simulink subsystem "SimscapePlantModels"  (R2023a)
settings: Solver=VariableStepAuto  StartTime=0.0  StopTime=10.0  RelTol=1e-3
undefined symbols (not defined in the file): AxlFL, AxlFR, AxlRL, AxlRR, EM1, EM2, EM3, EM4, PlntDCDCVoltInit, PlntTrnsfrCaseAxlSpdLock, PlntTrnsfrCaseTrqSplitRatio, ThrmBatt, ThrmBatt1, ThrmBatt2, ThrmBatt3, ThrmBatt4, ThrmEM, ThrmEM1, ThrmEM2, ThrmEM3, ThrmEM4, ThrmPwrE
libraries: fl_lib x30, nesl_utility_internal x13, sdl_lib x3, vehdynlibsens x1, nesl_utility x1
(part 2 of 2)

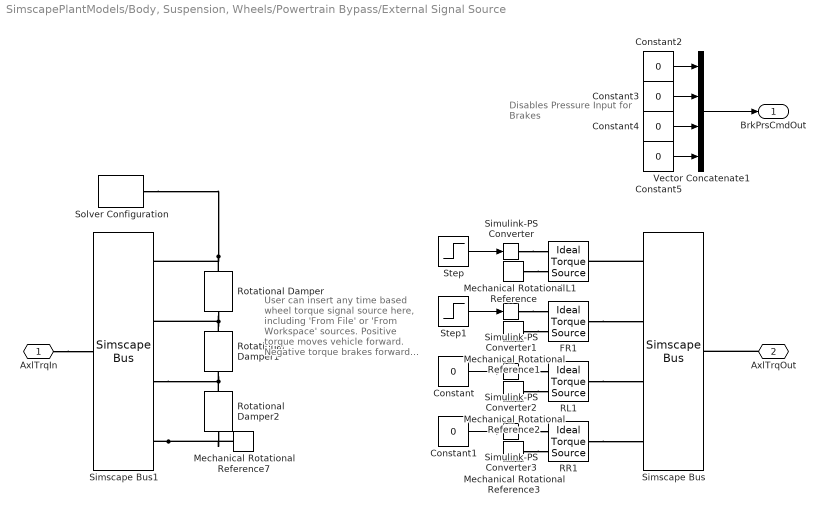
== system SimscapePlantModels/Body, Suspension, Wheels/Powertrain Bypass/External Signal Source ==
  note: User can insert any time based
      | wheel torque signal source here,
      | including 'From File' or 'From
      | Workspace' sources.
      |
      | Positive torque moves vehicle
      | forward.
      | Negative torque brakes forward
      | moving vehicle or moves vehicle
      | in reverse.
  note: Disables Pressure
      | Input for Brakes
  Constant{,1..5} (6 alike) : Constant  Value=0  SampleTime=-1
  FL1 : fl_lib/Mechanical/Mechanical Sources/Ideal Torque Source
  FR1 : fl_lib/Mechanical/Mechanical Sources/Ideal Torque Source
  Mechanical Rotational Reference{,1..3,7} (5 alike) : fl_lib/Mechanical/Rotational Elements/Mechanical Rotational Reference
  RL1 : fl_lib/Mechanical/Mechanical Sources/Ideal Torque Source
  RR1 : fl_lib/Mechanical/Mechanical Sources/Ideal Torque Source
  Rotational Damper : sdl_lib/Couplings & Drives/Springs & Dampers/Rotational Damper  D=1e5 N*m*s/rad  enable_faults=simscape.enum.onoff.off  b_fault=100 N*m*s/rad  temporal_fault=simscape.enum.onoff.off  fault_time=5 s  shock_fault=simscape.enum.onoff.off  acceleration_limit=100 rad/s^2  shock_limit=1  report_fault=simscape.enum.assert.action.none  thermal_port=simscape.enum.thermaleffects.omit  thermal_mass=50 kJ/K  temperature_specify=off  temperature_priority=High  temperature=300 K  temperature_nominal_specify=off  temperature_nominal_unit=K  temperature_nominal_value=1
  Rotational Damper1 : sdl_lib/Couplings & Drives/Springs & Dampers/Rotational Damper  D=1e5 N*m*s/rad  enable_faults=simscape.enum.onoff.off  b_fault=100 N*m*s/rad  temporal_fault=simscape.enum.onoff.off  fault_time=5 s  shock_fault=simscape.enum.onoff.off  acceleration_limit=100 rad/s^2  shock_limit=1  report_fault=simscape.enum.assert.action.none  thermal_port=simscape.enum.thermaleffects.omit  thermal_mass=50 kJ/K  temperature_specify=off  temperature_priority=High  temperature=300 K  temperature_nominal_specify=off  temperature_nominal_unit=K  temperature_nominal_value=1
  Rotational Damper2 : sdl_lib/Couplings & Drives/Springs & Dampers/Rotational Damper  D=1e5 N*m*s/rad  enable_faults=simscape.enum.onoff.off  b_fault=100 N*m*s/rad  temporal_fault=simscape.enum.onoff.off  fault_time=5 s  shock_fault=simscape.enum.onoff.off  acceleration_limit=100 rad/s^2  shock_limit=1  report_fault=simscape.enum.assert.action.none  thermal_port=simscape.enum.thermaleffects.omit  thermal_mass=50 kJ/K  temperature_specify=off  temperature_priority=High  temperature=300 K  temperature_nominal_specify=off  temperature_nominal_unit=K  temperature_nominal_value=1
  Simscape Bus : SimscapeBus  HierarchyStrings=AxlFL;AxlFR;AxlRL;AxlRR
  Simscape Bus1 : SimscapeBus  HierarchyStrings=AxlFL;AxlFR;AxlRL;AxlRR
  Simulink-PS Converter{,1..3} (4 alike) : nesl_utility_internal/Simulink-PS Converter  PhysicalDomain=network_engine_domain  SubClassName=ps_input  LeftPortType=input  RightPortType=output  PseudoPeriodic=off  Frequencies=[]  NoiseDistribution=none  NoiseParameters=[]  Unit=1  AffineConversion=off  FilteringAndDerivatives=provide  SimscapeFilterOrder=1  InputFilterTimeConstant=0.001  UdotUserProvided=0
  Solver Configuration : nesl_utility_internal/Solver Configuration  PhysicalDomain=network_engine_domain  SubClassName=solver  LeftPortType=input  RightPortType=generic  Tones=[]  Harmonics=[]  SimulateNoise=off  Profile=off  UseLocalSampling=off  EnableSwitchedLinearOptims=on  FrequencyDomain=off  UseCCode=off  RelTol=0.001  AbsTol=0.001  MinStep=1e-09  ToWorkspace=off  RevertToSquareIcSolve=off  NumHomotopyIterations=100  PhasorMode=off  PhasorModeNumHarmonics=1  ConsistencySolver=NEWTON_XTOL_AFTER_FTOL  IndexReductionMethod=DerivativeReplacement  DoDC=off  ResidualTolerance=1e-09  ConsistencyTolSource=GLOBAL  ConsistencyAbsTol=0.001  ConsistencyRelTol=0.001  ConsistencyTolFactor=0.001  UseLocalSolver=off  LocalSolverChoice=NE_BACKWARD_EULER_ADVANCER  ResolveIndetEquations=on  FunctionEvalNumThread=1  LocalSolverSampleTime=0.001  DoFixedCost=off  MaxNonlinIter=3  MaxModeIter=2  ComputeImpulses=off  ImpulseIterations=2  LinearAlgebra=auto  LinearAlgebraNumThread=0  EquationFormulation=NE_TIME_EF  DelaysMemoryBudget=1024  AutomaticFiltering=on  FilteringTimeConstant=0.001  PartitionStorageMethod=AS_NEEDED  PartitionMemoryBudget=1024  PartitionMethod=ROBUST
  Step : Step  After=100  SampleTime=0
  Step1 : Step  After=100  SampleTime=0
  Vector Concatenate1 : Concatenate  NumInputs=4
  AxlTrqIn : PMIOPort  Side=Left
  AxlTrqOut : PMIOPort  Port=2  Side=Right
  BrkPrsCmdOut : Outport
  wires:
  Constant2/1 -> Vector Concatenate1/1
  Constant3/1 -> Vector Concatenate1/2
  Constant4/1 -> Vector Concatenate1/3
  Vector Concatenate1/1 -> BrkPrsCmdOut/1
  Constant5/1 -> Vector Concatenate1/4
  Step1/1 -> Simulink-PS Converter1/1
  Step/1 -> Simulink-PS Converter/1
  Constant1/1 -> Simulink-PS Converter3/1
  Constant/1 -> Simulink-PS Converter2/1
  connections:
  Rotational Damper/LConn1 -- Simscape Bus1/LConn1 -- Solver Configuration/RConn1
  Rotational Damper2/LConn1 -- Simscape Bus1/LConn3 -- Rotational Damper1/RConn1
  Simscape Bus1/LConn4 -- Rotational Damper2/RConn1 -- Mechanical Rotational Reference7/LConn1
  Rotational Damper1/LConn1 -- Rotational Damper/RConn1 -- Simscape Bus1/LConn2
  Simulink-PS Converter3/RConn1 -- RR1/RConn1
  AxlTrqOut/RConn1 -- Simscape Bus/RConn1
  RR1/LConn1 -- Simscape Bus/LConn4
  Mechanical Rotational Reference1/LConn1 -- FR1/RConn2
  FR1/LConn1 -- Simscape Bus/LConn2
  AxlTrqIn/RConn1 -- Simscape Bus1/RConn1
  Simulink-PS Converter2/RConn1 -- RL1/RConn1
  RL1/LConn1 -- Simscape Bus/LConn3
  Mechanical Rotational Reference/LConn1 -- FL1/RConn2
  Simulink-PS Converter/RConn1 -- FL1/RConn1
  Mechanical Rotational Reference3/LConn1 -- RR1/RConn2
  Simscape Bus/LConn1 -- FL1/LConn1
  Simulink-PS Converter1/RConn1 -- FR1/RConn1
  Mechanical Rotational Reference2/LConn1 -- RL1/RConn2

== system SimscapePlantModels/Body, Suspension, Wheels/Powertrain Bypass/Pass Through ==
  BrkPrsCmdIn : Inport
  AxlTrqIn : PMIOPort  Side=Left
  AxlTrqOut : PMIOPort  Port=2  Side=Right
  BrkPrsCmdOut : Outport
  wires:
  BrkPrsCmdIn/1 -> BrkPrsCmdOut/1
  connections:
  AxlTrqOut/RConn1 -- AxlTrqIn/RConn1

== system SimscapePlantModels/Drivetrain/Drivetrain Layout/AxlTrqFL ==
  Ideal Torque Sensor : fl_lib/Mechanical/Mechanical Sensors/Ideal Torque Sensor
  PS-Simulink Converter : nesl_utility_internal/PS-Simulink Converter  PhysicalDomain=network_engine_domain  SubClassName=ps_output  LeftPortType=input  RightPortType=output  PseudoPeriodic=off  Frequencies=[]  VectorFormat=inherit  Unit=inherit  AffineConversion=off
  R : PMIOPort  Side=Left
  C : PMIOPort  Port=2  Side=Right
  Trq : Outport
  wires:
  PS-Simulink Converter/1 -> Trq/1
  connections:
  Ideal Torque Sensor/LConn1 -- R/RConn1
  Ideal Torque Sensor/RConn1 -- C/RConn1
  PS-Simulink Converter/LConn1 -- Ideal Torque Sensor/RConn2

== system SimscapePlantModels/Drivetrain/Drivetrain Layout/AxlTrqFR ==
  Ideal Torque Sensor : fl_lib/Mechanical/Mechanical Sensors/Ideal Torque Sensor
  PS-Simulink Converter : nesl_utility_internal/PS-Simulink Converter  PhysicalDomain=network_engine_domain  SubClassName=ps_output  LeftPortType=input  RightPortType=output  PseudoPeriodic=off  Frequencies=[]  VectorFormat=inherit  Unit=inherit  AffineConversion=off
  R : PMIOPort  Side=Left
  C : PMIOPort  Port=2  Side=Right
  Trq : Outport
  wires:
  PS-Simulink Converter/1 -> Trq/1
  connections:
  PS-Simulink Converter/LConn1 -- Ideal Torque Sensor/RConn2
  Ideal Torque Sensor/RConn1 -- C/RConn1
  Ideal Torque Sensor/LConn1 -- R/RConn1

== system SimscapePlantModels/Drivetrain/Drivetrain Layout/AxlTrqR ==
  Ideal Torque Sensor : fl_lib/Mechanical/Mechanical Sensors/Ideal Torque Sensor
  PS-Simulink Converter : nesl_utility_internal/PS-Simulink Converter  PhysicalDomain=network_engine_domain  SubClassName=ps_output  LeftPortType=input  RightPortType=output  PseudoPeriodic=off  Frequencies=[]  VectorFormat=inherit  Unit=inherit  AffineConversion=off
  R : PMIOPort  Side=Left
  C : PMIOPort  Port=2  Side=Right
  Trq : Outport
  wires:
  PS-Simulink Converter/1 -> Trq/1
  connections:
  PS-Simulink Converter/LConn1 -- Ideal Torque Sensor/RConn2
  Ideal Torque Sensor/RConn1 -- C/RConn1
  Ideal Torque Sensor/LConn1 -- R/RConn1

== system SimscapePlantModels/Drivetrain/Drivetrain Layout/AxlTrqRL ==
  Ideal Torque Sensor : fl_lib/Mechanical/Mechanical Sensors/Ideal Torque Sensor
  PS-Simulink Converter : nesl_utility_internal/PS-Simulink Converter  PhysicalDomain=network_engine_domain  SubClassName=ps_output  LeftPortType=input  RightPortType=output  PseudoPeriodic=off  Frequencies=[]  VectorFormat=inherit  Unit=inherit  AffineConversion=off
  R : PMIOPort  Side=Left
  C : PMIOPort  Port=2  Side=Right
  Trq : Outport
  wires:
  PS-Simulink Converter/1 -> Trq/1
  connections:
  Ideal Torque Sensor/LConn1 -- R/RConn1
  Ideal Torque Sensor/RConn1 -- C/RConn1
  PS-Simulink Converter/LConn1 -- Ideal Torque Sensor/RConn2

== system SimscapePlantModels/Drivetrain/Drivetrain Layout/Axle Interconnect ==
  SplitRatio : Inport
  Lockup : Inport  Port=2
  No Interconnect : Subsystem  VariantControl=No Interconnect
  Transfer Case : Subsystem  VariantControl=Transfer Case  ReferencedSubsystem=TransferCaseSSC
  FrntDiffrntlTrq : PMIOPort  Side=Left
  DriveshftTrq : PMIOPort  Port=2  Side=Left
  RearDiffrntlTrq : PMIOPort  Port=3  Side=Left

== system SimscapePlantModels/Drivetrain/Drivetrain Layout/DriveshftTrq Routing ==
  Four Actuator AWD : Subsystem  VariantControl=Four Actuator AWD  ReferencedSubsystem=FourActuatorAWDSSC
  One Actuator AWD : Subsystem  VariantControl=One Actuator AWD  ReferencedSubsystem=OneActuatorAWDSSC
  One Actuator FWD : Subsystem  VariantControl=One Actuator FWD  ReferencedSubsystem=OneActuatorFWDSSC
  One Actuator RWD : Subsystem  VariantControl=One Actuator RWD  ReferencedSubsystem=OneActuatorRWDSSC
  Three Actuator AWD Dual EM Front : Subsystem  VariantControl=Three Actuator AWD Dual EM Front  ReferencedSubsystem=ThreeActuatorAWD2EMFrontSSC
  Three Actuator AWD Dual EM Rear : Subsystem  VariantControl=Three Actuator AWD Dual EM Rear  ReferencedSubsystem=ThreeActuatorAWD2EMRearSSC
  Two Actuator AWD : Subsystem  VariantControl=Two Actuator AWD  ReferencedSubsystem=TwoActuatorAWDSSC
  DriveshftTrq : PMIOPort  Side=Left
  FrntDiffrntlTrq : PMIOPort  Port=2  Side=Right
  TrnsfrCaseFrntTrq : PMIOPort  Port=3  Side=Right
  TrnsfrCaseTrq : PMIOPort  Port=4  Side=Right
  TrnsfrCaseRearTrq : PMIOPort  Port=5  Side=Right
  RearDiffrntlTrq : PMIOPort  Port=6  Side=Right
  DriveshftSpd : Outport  VectorParamsAs1DForOutWhenUnconnected=off

== system SimscapePlantModels/Drivetrain/Drivetrain Layout/Front Axle ==
  Prs1 : Inport
  Prs2 : Inport  Port=2
  Dual EM Drive Front : Subsystem  VariantControl=Dual EM Drive Front  ReferencedSubsystem=DualEMDriveFrontSSC
  Limited Slip Differential : Subsystem  VariantControl=Limited Slip Differential  ReferencedSubsystem=LimitedSlipDifferentialSSC
  No Differential : Subsystem  VariantControl=No Differential  ReferencedSubsystem=NoDifferentialFrontSSC
  Open Differential : Subsystem  VariantControl=Open Differential  ReferencedSubsystem=OpenDifferentialSSC
  DriveshftTrq : PMIOPort  Side=Left
  AxlTrqFL : PMIOPort  Port=2  Side=Right
  AxlTrqFR : PMIOPort  Port=3  Side=Right
  Info : Outport
  DriveshftSpd : Outport  Port=2
  Axl1Spd : Outport  Port=3
  Axl2Spd : Outport  Port=4

== system SimscapePlantModels/Drivetrain/Drivetrain Layout/Rear Axle ==
  Prs1 : Inport
  Prs2 : Inport  Port=2
  Dual EM Rear 3EM : Subsystem  VariantControl=Dual EM Rear 3EM  ReferencedSubsystem=DualEMDriveRear3EMSSC
  Dual EM Rear 4EM : Subsystem  VariantControl=Dual EM Rear 4EM  ReferencedSubsystem=DualEMDriveRear4EMSSC
  Limited Slip Differential : Subsystem  VariantControl=Limited Slip Differential  ReferencedSubsystem=LimitedSlipDifferential2SSC
  No Differential : Subsystem  VariantControl=No Differential  ReferencedSubsystem=NoDifferentialRearSSC
  Open Differential : Subsystem  VariantControl=Open Differential  ReferencedSubsystem=OpenDifferential2SSC
  DriveshftTrq : PMIOPort  Side=Left
  AxlTrqRL : PMIOPort  Port=2  Side=Right
  AxlTrqRR : PMIOPort  Port=3  Side=Right
  Info : Outport
  DriveshftSpd : Outport  Port=2
  Axl1Spd : Outport  Port=3
  Axl2Spd : Outport  Port=4

== system SimscapePlantModels/Drivetrain/Transmission and Actuators/Conventional Vehicle ==
  note: Copyright 2021 The MathWorks, Inc.
  GearCmd : Inport
  Bus Creator : BusCreator  Inputs=3
  Constant : Constant  Value=0  SampleTime=-1
  Inertia1 : fl_lib/Mechanical/Rotational Elements/Inertia  inertia=PlntEngInertia kg*m^2  num_ports=foundation.enum.numPorts2.two  w_specify=off  w_priority=High  w=0 rad/s  w_nominal_specify=off  w_nominal_unit=rad/s  w_nominal_value=1  t_specify=off  t_priority=None  t=0 N*m  t_nominal_specify=off  t_nominal_unit=N*m  t_nominal_value=1
      settings: InternalSimscapePortConfiguration="{\"Bottom\":[],\"Left\":[{\"id\":\"I\",\"label\":\"\",\"type\":\"foundation.mechanical.rotational.rotational\"}],\"Right\":[{\"id\":\"J\",\"label\":\"\",\"type\":\"foundation.mechanical.rotational.rotational\"}],\"Top\":[]}"
  Simscape Bus1 : SimscapeBus  HierarchyStrings=DriveshftTrq1
  Spd Sensor : Subsystem
  Transmission : Subsystem  Variant=on  VariantControlMode=label  VariantControl=1  LabelModeActiveChoice=Ideal Fixed Gear Transmission
  DriveshftTrq : PMIOPort  Side=Right
  EngTrq : PMIOPort  Port=2  Side=Left
  Info : Outport
  EngSpd : Outport  Port=2
  wires:
  Constant/1 -> Bus Creator/1  "Cltch1State"
  Transmission/2(Info) -> Bus Creator/3  "TransInfo"
  Transmission/1(Cltch2State) -> Bus Creator/2  "Cltch2State"
  GearCmd/1 -> Transmission/1(GearCmd)
  Bus Creator/1 -> Info/1
  Spd Sensor/1(w) -> EngSpd/1
  connections:
  DriveshftTrq/RConn1 -- Simscape Bus1/RConn1
  Inertia1/LConn1 -- Transmission/LConn1
  Spd Sensor/LConn1 -- EngTrq/RConn1 -- Inertia1/RConn1
  Simscape Bus1/LConn1 -- Transmission/RConn1

== system SimscapePlantModels/Electrical System/Electrical System/Battery System ==
  P_Acc : Inport
  BMS : Inport  Port=2
  AmbTemp : Inport  Port=3
  Detailed Battery : Subsystem  VariantControl=Detailed Battery  ReferencedSubsystem=DetailedBatteryModel
  Mapped Battery : Subsystem  VariantControl=Mapped Battery  ReferencedSubsystem=BatteryMappedSSC
  + : PMIOPort  Side=Right
  - : PMIOPort  Port=2  Side=Right
  ThrmBatt : PMIOPort  Port=3  Side=Right
  BattSoc : Outport  VectorParamsAs1DForOutWhenUnconnected=off
  BattVolt : Outport  Port=2  VectorParamsAs1DForOutWhenUnconnected=off
  BattCurr : Outport  Port=3  VectorParamsAs1DForOutWhenUnconnected=off
  BMSSensors : Outport  Port=4  VectorParamsAs1DForOutWhenUnconnected=off

== system SimscapePlantModels/Electrical System/Electrical System/DC-DC Converter ==
  DC-DC Converter : Subsystem  VariantControl=DC-DC Converter  ReferencedSubsystem=DCDCConverterSSC
  No DC-DC Converter : Subsystem  VariantControl=No DC-DC Converter  ReferencedSubsystem=NoDCDCConverterSSC
  1+ : PMIOPort  Side=Left
  2+ : PMIOPort  Port=2  Side=Right
  1- : PMIOPort  Port=3  Side=Left
  2- : PMIOPort  Port=4  Side=Right
  H : PMIOPort  Port=5  Side=Right
  Vref : PMIOPort  Port=6  Side=Left

== system SimscapePlantModels/Electrical System/Electrical System/Electric Machines ==
  EMTrqCmd : Inport
  1EM : Subsystem  VariantControl=1EM
  2EM : Subsystem  VariantControl=2EM
  3EM : Subsystem  VariantControl=3EM
  4EM : Subsystem  VariantControl=4EM
  + : PMIOPort  Side=Left
  EM : PMIOPort  Port=2  Side=Right
  - : PMIOPort  Port=3  Side=Left
  ThrmEM : PMIOPort  Port=4  Side=Right
  EMTrq : Outport
  EMPwrElec : Outport  Port=2

== system SimscapePlantModels/Electrical System/Electrical System 1EM/Battery System ==
  note: 1) Add Subsystem or Model blocks as valid variant choices.
      | 2) You cannot connect blocks at this level. At simulation, connectivity is automatically
      | determined, based on the active variant and port name matching.
  P_Acc : Inport
  BMS : Inport  Port=2
  AmbTemp : Inport  Port=3
  Detailed Battery : Subsystem  VariantControl=Detailed Battery  ReferencedSubsystem=DetailedBatteryModel
  Mapped Battery : Subsystem  VariantControl=Mapped Battery  ReferencedSubsystem=BatteryMappedSSC
  + : PMIOPort  Side=Right
  - : PMIOPort  Port=2  Side=Right
  BattSoc : Outport  VectorParamsAs1DForOutWhenUnconnected=off
  BattVolt : Outport  Port=2  VectorParamsAs1DForOutWhenUnconnected=off
  BattCurr : Outport  Port=3  VectorParamsAs1DForOutWhenUnconnected=off
  BMSSensors : Outport  Port=4  VectorParamsAs1DForOutWhenUnconnected=off

== system SimscapePlantModels/Electrical System/Electrical System 1EM/DC-DC Converter ==
  DC-DC Converter : Subsystem  VariantControl=DC-DC Converter  ReferencedSubsystem=DCDCConverterSSC
  No DC-DC Converter : Subsystem  VariantControl=No DC-DC Converter  ReferencedSubsystem=NoDCDCConverterSSC
  1+ : PMIOPort  Side=Left
  2+ : PMIOPort  Port=2  Side=Right
  1- : PMIOPort  Port=3  Side=Left
  2- : PMIOPort  Port=4  Side=Right
  H : PMIOPort  Port=5  Side=Right
  Vref : PMIOPort  Port=6  Side=Left

== system SimscapePlantModels/Electrical System/Electrical System 1EM/Electric Machine 1 ==
  EMTrqCmd : Inport
  Mapped EM : Subsystem  VariantControl=Mapped EM  ReferencedSubsystem=ElectricMachine1SSC
  + : PMIOPort  Side=Left
  - : PMIOPort  Port=2  Side=Left
  R : PMIOPort  Port=3  Side=Right
  H : PMIOPort  Port=4  Side=Right
  EMTrq : Outport  VectorParamsAs1DForOutWhenUnconnected=off
  EMPwrElec : Outport  Port=2  VectorParamsAs1DForOutWhenUnconnected=off

== system SimscapePlantModels/Electrical System/Electrical System 2EM/Battery System ==
  note: 1) Add Subsystem or Model blocks as valid variant choices.
      | 2) You cannot connect blocks at this level. At simulation, connectivity is automatically
      | determined, based on the active variant and port name matching.
  P_Acc : Inport
  BMS : Inport  Port=2
  AmbTemp : Inport  Port=3
  Detailed Battery : Subsystem  VariantControl=Detailed Battery  ReferencedSubsystem=DetailedBatteryModel
  Mapped Battery : Subsystem  VariantControl=Mapped Battery  ReferencedSubsystem=BatteryMappedSSC
  + : PMIOPort  Side=Right
  - : PMIOPort  Port=2  Side=Right
  BattSoc : Outport  VectorParamsAs1DForOutWhenUnconnected=off
  BattVolt : Outport  Port=2  VectorParamsAs1DForOutWhenUnconnected=off
  BattCurr : Outport  Port=3  VectorParamsAs1DForOutWhenUnconnected=off
  BMSSensors : Outport  Port=4  VectorParamsAs1DForOutWhenUnconnected=off

== system SimscapePlantModels/Electrical System/Electrical System 2EM/DC-DC Converter ==
  DC-DC Converter : Subsystem  VariantControl=DC-DC Converter  ReferencedSubsystem=DCDCConverterSSC
  No DC-DC Converter : Subsystem  VariantControl=No DC-DC Converter  ReferencedSubsystem=NoDCDCConverterSSC
  1+ : PMIOPort  Side=Left
  2+ : PMIOPort  Port=2  Side=Right
  1- : PMIOPort  Port=3  Side=Left
  2- : PMIOPort  Port=4  Side=Right
  H : PMIOPort  Port=5  Side=Right
  Vref : PMIOPort  Port=6  Side=Left

== system SimscapePlantModels/Electrical System/Electrical System 2EM/Electric Machine 1 ==
  EMTrqCmd : Inport
  Mapped EM : Subsystem  VariantControl=Mapped EM  ReferencedSubsystem=ElectricMachine1SSC
  + : PMIOPort  Side=Left
  - : PMIOPort  Port=2  Side=Left
  R : PMIOPort  Port=3  Side=Right
  H : PMIOPort  Port=4  Side=Right
  EMTrq : Outport  VectorParamsAs1DForOutWhenUnconnected=off
  EMPwrElec : Outport  Port=2  VectorParamsAs1DForOutWhenUnconnected=off

== system SimscapePlantModels/Electrical System/Electrical System 2EM/Electric Machine 2 ==
  EMTrqCmd : Inport
  Mapped EM : Subsystem  VariantControl=Mapped EM  ReferencedSubsystem=ElectricMachine2SSC
  + : PMIOPort  Side=Left
  - : PMIOPort  Port=2  Side=Left
  R : PMIOPort  Port=3  Side=Right
  H : PMIOPort  Port=4  Side=Right
  EMTrq : Outport  VectorParamsAs1DForOutWhenUnconnected=off
  EMPwrElec : Outport  Port=2  VectorParamsAs1DForOutWhenUnconnected=off

== system SimscapePlantModels/Sensors/Sensors/IMU Sensor ==
  VehFdbk : Inport
  Bus Creator1 : BusCreator  Inputs=2
  Bus Selector : BusSelector  OutputSignals=BdyFrm.Cg.Acc.ax,BdyFrm.Cg.Acc.ay,BdyFrm.Cg.Acc.az  OutputAsBus=on
  Bus Selector1 : BusSelector  OutputSignals=BdyFrm.Cg.AngVel.p,BdyFrm.Cg.AngVel.q,BdyFrm.Cg.AngVel.r  OutputAsBus=on
  Bus Selector2 : BusSelector  OutputSignals=BdyFrm.Cg.AngAcc.pdot,BdyFrm.Cg.AngAcc.qdot,BdyFrm.Cg.AngAcc.rdot  OutputAsBus=on
  Bus to Vector : BusToVector
  Bus to Vector1 : BusToVector
  Bus to Vector2 : BusToVector
  Constant : Constant  Value=[0,0,0]
  Constant1 : Constant  Value=[0,0,9.81]
  Three-axis Inertial Measurement Unit : vehdynlibsens/Three-axis Inertial Measurement Unit  units=Metric (MKS)  imu=[0 0 0]  i_Ts=0  dtype_a=off  w_a=190  z_a=0.707  a_sf_cc=[1 0 0; 0 1 0; 0 0 1]  a_bias=[0 0 0]  a_sat="[-inf  -inf  -inf  inf inf inf]"  dtype_g=off  w_g=190  z_g=0.707  g_sf_cc=[1 0 0; 0 1 0; 0 0 1]  g_bias=[0 0 0]  g_sens=[0 0 0]  g_sat="[-inf  -inf  -inf  inf inf inf]"  i_rand=on  i_seeds=[23093 23094 23095 23096 23097 23098]  i_pow=[0.001 0.001 0.001 0.0001 0.0001 0.0001]  aMode=2
  Unit Conversion : UnitConversion
  IMU : Outport
  wires:
  VehFdbk/1 -> Bus Selector/1, Bus Selector1/1, Bus Selector2/1
  Constant1/1 -> Three-axis Inertial Measurement Unit/5
  Bus to Vector/1 -> Unit Conversion/1
  Bus Selector1/1 -> Bus to Vector1/1
  Bus to Vector1/1 -> Three-axis Inertial Measurement Unit/2
  Bus Selector/1 -> Bus to Vector/1
  Bus to Vector2/1 -> Three-axis Inertial Measurement Unit/3
  Three-axis Inertial Measurement Unit/1 -> Bus Creator1/1  "Acc"
  Bus Creator1/1 -> IMU/1  "IMU"
  Bus Selector2/1 -> Bus to Vector2/1
  Constant/1 -> Three-axis Inertial Measurement Unit/4
  Three-axis Inertial Measurement Unit/2 -> Bus Creator1/2  "pqr"
  Unit Conversion/1 -> Three-axis Inertial Measurement Unit/1

== system SimscapePlantModels/Sensors/Sensors/No IMU Sensor ==
  VehFdbk : Inport
  Bus Creator1 : BusCreator  Inputs=2
  Constant : Constant  Value=zeros(3,1)
  Constant1 : Constant  Value=zeros(3,1)
  Terminator : Terminator
  IMU : Outport
  wires:
  VehFdbk/1 -> Terminator/1
  Constant1/1 -> Bus Creator1/2  "pqr"
  Bus Creator1/1 -> IMU/1  "IMU"
  Constant/1 -> Bus Creator1/1  "Acc"

== system SimscapePlantModels/Thermal/Electrical Cooling/No Thermal Effect ==
  BMSSensors : Inport
  VehBody : Inport  Port=2
  Constant : Constant  Value=0  SampleTime=-1
  Constant1 : Constant  Value=0  SampleTime=-1
  Simscape Bus : SimscapeBus  HierarchyStrings=ThrmEM;ThrmBatt;ThrmPwrE
  Simscape Bus1 : SimscapeBus  HierarchyStrings=ThrmEM4;ThrmEM3;ThrmEM2;ThrmEM1
  Simscape Bus2 : SimscapeBus  HierarchyStrings=ThrmBatt4;ThrmBatt3;ThrmBatt2;ThrmBatt1
  Simscape Bus3 : SimscapeBus  HierarchyStrings=ThrmPwrE1
  Temperature Source{,1..8} (9 alike) : fl_lib/Thermal/Thermal Sources/Temperature Source  temperature=EnvAirTemp K
  Terminator : Terminator
  Terminator1 : Terminator
  ThrmElec : PMIOPort  Side=Left
  Out Bus Element : Outport  PortName=Thermal  Element=EPumpPwr
  Out Bus Element1 : Outport  PortName=Thermal  Element=CoolTemp
  wires:
  VehBody/1 -> Terminator1/1
  BMSSensors/1 -> Terminator/1
  Constant/1 -> Out Bus Element/1
  Constant1/1 -> Out Bus Element1/1
  connections:
  Temperature Source3/LConn1 -- Simscape Bus1/LConn4
  Simscape Bus/LConn2 -- Simscape Bus2/RConn1
  Simscape Bus1/RConn1 -- Simscape Bus/LConn1
  ThrmElec/RConn1 -- Simscape Bus/RConn1
  Temperature Source7/LConn1 -- Simscape Bus2/LConn4
  Temperature Source6/LConn1 -- Simscape Bus2/LConn3
  Temperature Source4/LConn1 -- Simscape Bus2/LConn1
  Temperature Source5/LConn1 -- Simscape Bus2/LConn2
  Temperature Source2/LConn1 -- Simscape Bus1/LConn3
  Temperature Source1/LConn1 -- Simscape Bus1/LConn2
  Temperature Source/LConn1 -- Simscape Bus1/LConn1
  Temperature Source8/LConn1 -- Simscape Bus3/LConn1
  Simscape Bus/LConn3 -- Simscape Bus3/RConn1

== system SimscapePlantModels/Drivetrain/Drivetrain Layout/Axle Interconnect/No Interconnect ==

== system SimscapePlantModels/Drivetrain/Transmission and Actuators/Conventional Vehicle/Spd Sensor ==
  Ideal Rotational Motion Sensor : fl_lib/Mechanical/Mechanical Sensors/Ideal Rotational Motion Sensor  reference=foundation.enum.MeasurementReference.difference  acceleration_port=false  velocity_port=true  position_port=true  wrap_angle=simscape.enum.onoff.off  offset=0 rad
  Mechanical Rotational Reference : fl_lib/Mechanical/Rotational Elements/Mechanical Rotational Reference
  PS-Simulink Converter : nesl_utility_internal/PS-Simulink Converter  PhysicalDomain=network_engine_domain  SubClassName=ps_output  LeftPortType=input  RightPortType=output  PseudoPeriodic=off  Frequencies=[]  VectorFormat=inherit  Unit=inherit  AffineConversion=off
  R : PMIOPort  Side=Left
  w : Outport
  wires:
  PS-Simulink Converter/1 -> w/1
  connections:
  PS-Simulink Converter/LConn1 -- Ideal Rotational Motion Sensor/RConn2
  Ideal Rotational Motion Sensor/LConn1 -- R/RConn1
  Ideal Rotational Motion Sensor/RConn1 -- Mechanical Rotational Reference/LConn1

== system SimscapePlantModels/Drivetrain/Transmission and Actuators/Conventional Vehicle/Transmission ==
  GearCmd : Inport
  Automatic Transmission With Torque Converter : Subsystem  VariantControl=Automatic Transmission With Torque Converter  ReferencedSubsystem=AutomaticTransmissionWithTorqueConverterSSC
  Ideal Fixed Gear Transmission : Subsystem  VariantControl=Ideal Fixed Gear Transmission  ReferencedSubsystem=IdealFixedGearTransmissionSSC
  EngTrq : PMIOPort  Side=Left
  DriveshftTrq : PMIOPort  Port=2  Side=Right
  Cltch2State : Outport
  Info : Outport  Port=2

== system SimscapePlantModels/Electrical System/Electrical System/Electric Machines/1EM ==
  EMTrqCmd : Inport
  Electric Machine 1 : Subsystem  Variant=on  VariantControlMode=label  LabelModeActiveChoice=Mapped EM
  Simscape Bus : SimscapeBus  HierarchyStrings=EM1
  Simscape Bus1 : SimscapeBus  HierarchyStrings=ThrmEM1
  + : PMIOPort  Side=Left
  EM : PMIOPort  Port=2  Side=Right
  - : PMIOPort  Port=3  Side=Left
  ThrmEM : PMIOPort  Port=4  Side=Right
  EMTrq : Outport
  EMPwrElec : Outport  Port=2
  wires:
  EMTrqCmd/1 -> Electric Machine 1/1(EMTrqCmd)
  Electric Machine 1/2(EMPwrElec) -> EMPwrElec/1  "EMPwrElec"
  Electric Machine 1/1(EMTrq) -> EMTrq/1  "EMTrq"
  connections:
  Simscape Bus/RConn1 -- EM/RConn1
  -/RConn1 -- Electric Machine 1/LConn2
  +/RConn1 -- Electric Machine 1/LConn1
  Electric Machine 1/RConn1 -- Simscape Bus/LConn1
  ThrmEM/RConn1 -- Simscape Bus1/RConn1
  Simscape Bus1/LConn1 -- Electric Machine 1/RConn2

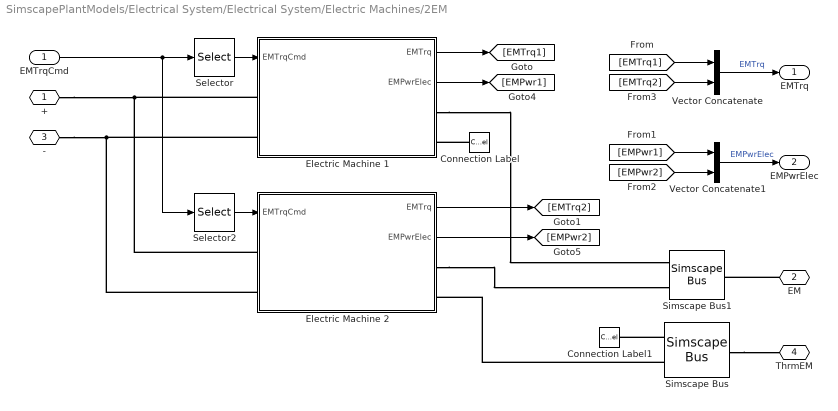
== system SimscapePlantModels/Electrical System/Electrical System/Electric Machines/2EM ==
  EMTrqCmd : Inport
  Connection Label : ConnectionLabel  Label=H1
  Connection Label1 : ConnectionLabel  Label=H1
  Electric Machine 1 : Subsystem  Variant=on  VariantControlMode=label  LabelModeActiveChoice=Mapped EM
  Electric Machine 2 : Subsystem  Variant=on  VariantControlMode=label  LabelModeActiveChoice=Mapped EM
  Selector : Selector  InputPortWidth=2  IndexOptions=Index vector (dialog)  Indices=[1]  OutputSizes=1
  Selector2 : Selector  InputPortWidth=2  IndexOptions=Index vector (dialog)  Indices=[2]  OutputSizes=1
  Simscape Bus : SimscapeBus  HierarchyStrings=ThrmEM1;ThrmEM2
  Simscape Bus1 : SimscapeBus  HierarchyStrings=EM1;EM2
  Vector Concatenate : Concatenate
  Vector Concatenate1 : Concatenate
  + : PMIOPort  Side=Left
  EM : PMIOPort  Port=2  Side=Right
  - : PMIOPort  Port=3  Side=Left
  ThrmEM : PMIOPort  Port=4  Side=Right
  EMTrq : Outport
  EMPwrElec : Outport  Port=2
  wires:
  [EMPwr2] -> Vector Concatenate1/2
  Electric Machine 2/2(EMPwrElec) -> [EMPwr2]
  [EMPwr1] -> Vector Concatenate1/1
  Electric Machine 1/2(EMPwrElec) -> [EMPwr1]
  Electric Machine 2/1(EMTrq) -> [EMTrq2]
  [EMTrq2] -> Vector Concatenate/2
  [EMTrq1] -> Vector Concatenate/1
  Electric Machine 1/1(EMTrq) -> [EMTrq1]
  Selector2/1 -> Electric Machine 2/1(EMTrqCmd)
  Vector Concatenate1/1 -> EMPwrElec/1  "EMPwrElec"
  Vector Concatenate/1 -> EMTrq/1  "EMTrq"
  Selector/1 -> Electric Machine 1/1(EMTrqCmd)
  EMTrqCmd/1 -> Selector/1, Selector2/1
  connections:
  EM/RConn1 -- Simscape Bus1/RConn1
  Electric Machine 2/RConn1 -- Simscape Bus1/LConn2
  Electric Machine 1/RConn1 -- Simscape Bus1/LConn1
  Electric Machine 2/LConn1 -- Electric Machine 1/LConn1 -- +/RConn1
  Electric Machine 2/LConn2 -- Electric Machine 1/LConn2 -- -/RConn1
  Simscape Bus/RConn1 -- ThrmEM/RConn1
  Connection Label/LConn1 -- Electric Machine 1/RConn2
  Simscape Bus/LConn1 -- Connection Label1/LConn1
  Simscape Bus/LConn2 -- Electric Machine 2/RConn2

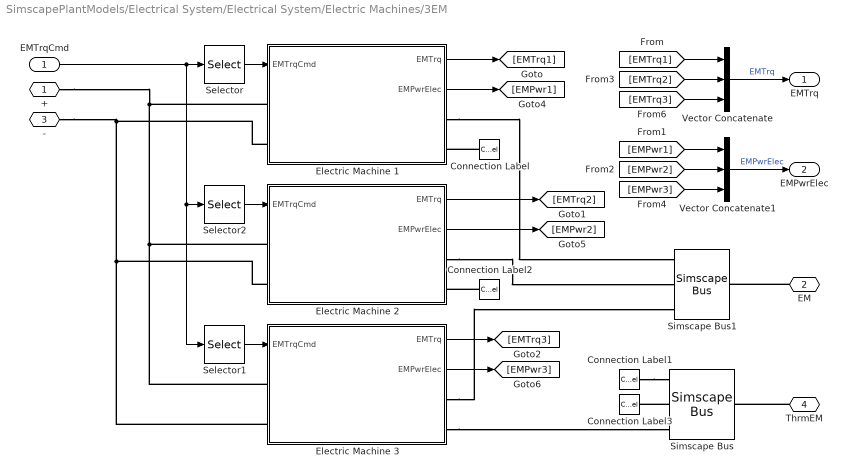
== system SimscapePlantModels/Electrical System/Electrical System/Electric Machines/3EM ==
  EMTrqCmd : Inport
  Connection Label : ConnectionLabel  Label=H1
  Connection Label1 : ConnectionLabel  Label=H1
  Connection Label2 : ConnectionLabel  Label=H2
  Connection Label3 : ConnectionLabel  Label=H2
  Electric Machine 1 : Subsystem  Variant=on  VariantControlMode=label  LabelModeActiveChoice=Mapped EM
  Electric Machine 2 : Subsystem  Variant=on  VariantControlMode=label  LabelModeActiveChoice=Mapped EM
  Electric Machine 3 : Subsystem  Variant=on  VariantControlMode=label  LabelModeActiveChoice=Mapped EM
  Selector : Selector  InputPortWidth=3  IndexOptions=Index vector (dialog)  Indices=[1]  OutputSizes=1
  Selector1 : Selector  InputPortWidth=3  IndexOptions=Index vector (dialog)  Indices=[3]  OutputSizes=1
  Selector2 : Selector  InputPortWidth=3  IndexOptions=Index vector (dialog)  Indices=[2]  OutputSizes=1
  Simscape Bus : SimscapeBus  HierarchyStrings=ThrmEM1;ThrmEM2;ThrmEM3
  Simscape Bus1 : SimscapeBus  HierarchyStrings=EM1;EM2;EM3
  Vector Concatenate : Concatenate  NumInputs=3
  Vector Concatenate1 : Concatenate  NumInputs=3
  + : PMIOPort  Side=Left
  EM : PMIOPort  Port=2  Side=Right
  - : PMIOPort  Port=3  Side=Left
  ThrmEM : PMIOPort  Port=4  Side=Right
  EMTrq : Outport
  EMPwrElec : Outport  Port=2
  wires:
  [EMPwr3] -> Vector Concatenate1/3
  Electric Machine 3/2(EMPwrElec) -> [EMPwr3]
  [EMPwr2] -> Vector Concatenate1/2
  Electric Machine 2/2(EMPwrElec) -> [EMPwr2]
  [EMPwr1] -> Vector Concatenate1/1
  Electric Machine 1/2(EMPwrElec) -> [EMPwr1]
  Electric Machine 3/1(EMTrq) -> [EMTrq3]
  Electric Machine 2/1(EMTrq) -> [EMTrq2]
  [EMTrq3] -> Vector Concatenate/3
  [EMTrq2] -> Vector Concatenate/2
  [EMTrq1] -> Vector Concatenate/1
  Electric Machine 1/1(EMTrq) -> [EMTrq1]
  Selector1/1 -> Electric Machine 3/1(EMTrqCmd)
  Selector2/1 -> Electric Machine 2/1(EMTrqCmd)
  Vector Concatenate1/1 -> EMPwrElec/1  "EMPwrElec"
  Vector Concatenate/1 -> EMTrq/1  "EMTrq"
  EMTrqCmd/1 -> Selector1/1, Selector2/1, Selector/1
  Selector/1 -> Electric Machine 1/1(EMTrqCmd)
  connections:
  Electric Machine 3/RConn1 -- Simscape Bus1/LConn3
  EM/RConn1 -- Simscape Bus1/RConn1
  Electric Machine 2/RConn1 -- Simscape Bus1/LConn2
  Electric Machine 1/RConn1 -- Simscape Bus1/LConn1
  Electric Machine 3/LConn1 -- +/RConn1 -- Electric Machine 1/LConn1 -- Electric Machine 2/LConn1
  Electric Machine 3/LConn2 -- -/RConn1 -- Electric Machine 1/LConn2 -- Electric Machine 2/LConn2
  Connection Label1/LConn1 -- Simscape Bus/LConn1
  Simscape Bus/LConn2 -- Connection Label3/LConn1
  ThrmEM/RConn1 -- Simscape Bus/RConn1
  Connection Label/LConn1 -- Electric Machine 1/RConn2
  Connection Label2/LConn1 -- Electric Machine 2/RConn2
  Electric Machine 3/RConn2 -- Simscape Bus/LConn3

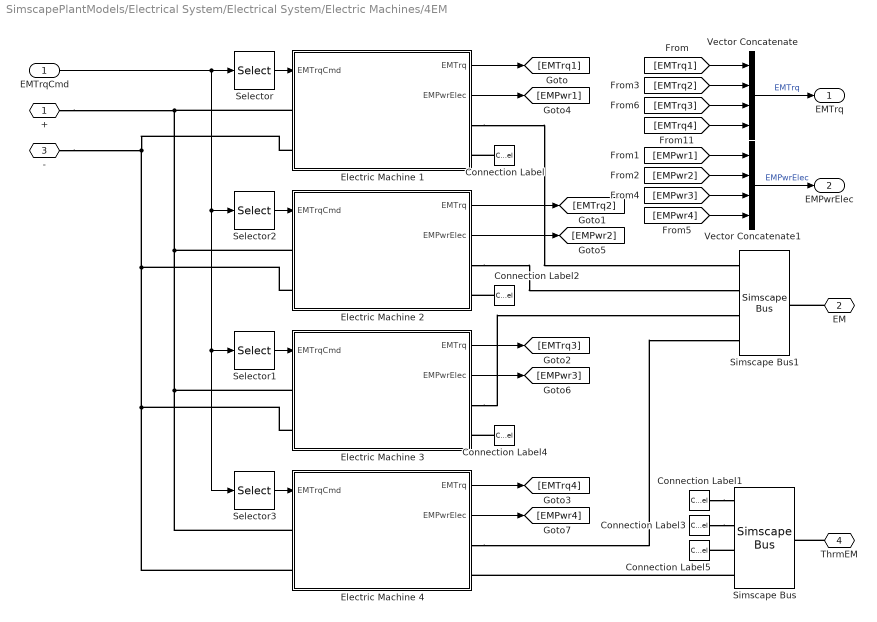
== system SimscapePlantModels/Electrical System/Electrical System/Electric Machines/4EM ==
  EMTrqCmd : Inport
  Connection Label : ConnectionLabel  Label=H1
  Connection Label1 : ConnectionLabel  Label=H1
  Connection Label2 : ConnectionLabel  Label=H2
  Connection Label3 : ConnectionLabel  Label=H2
  Connection Label4 : ConnectionLabel  Label=H3
  Connection Label5 : ConnectionLabel  Label=H3
  Electric Machine 1 : Subsystem  Variant=on  VariantControlMode=label  LabelModeActiveChoice=Mapped EM
  Electric Machine 2 : Subsystem  Variant=on  VariantControlMode=label  LabelModeActiveChoice=Mapped EM
  Electric Machine 3 : Subsystem  Variant=on  VariantControlMode=label  LabelModeActiveChoice=Mapped EM
  Electric Machine 4 : Subsystem  Variant=on  VariantControlMode=label  LabelModeActiveChoice=Mapped EM
  Selector : Selector  InputPortWidth=4  IndexOptions=Index vector (dialog)  Indices=[1]  OutputSizes=1
  Selector1 : Selector  InputPortWidth=4  IndexOptions=Index vector (dialog)  Indices=[3]  OutputSizes=1
  Selector2 : Selector  InputPortWidth=4  IndexOptions=Index vector (dialog)  Indices=[2]  OutputSizes=1
  Selector3 : Selector  InputPortWidth=4  IndexOptions=Index vector (dialog)  Indices=[4]  OutputSizes=1
  Simscape Bus : SimscapeBus  HierarchyStrings=ThrmEM1;ThrmEM2;ThrmEM3;ThrmEM4
  Simscape Bus1 : SimscapeBus  HierarchyStrings=EM1;EM2;EM3;EM4
  Vector Concatenate : Concatenate  NumInputs=4
  Vector Concatenate1 : Concatenate  NumInputs=4
  + : PMIOPort  Side=Left
  EM : PMIOPort  Port=2  Side=Right
  - : PMIOPort  Port=3  Side=Left
  ThrmEM : PMIOPort  Port=4  Side=Right
  EMTrq : Outport
  EMPwrElec : Outport  Port=2
  wires:
  [EMPwr4] -> Vector Concatenate1/4
  Electric Machine 4/2(EMPwrElec) -> [EMPwr4]
  [EMPwr3] -> Vector Concatenate1/3
  Electric Machine 3/2(EMPwrElec) -> [EMPwr3]
  [EMPwr2] -> Vector Concatenate1/2
  Electric Machine 2/2(EMPwrElec) -> [EMPwr2]
  [EMPwr1] -> Vector Concatenate1/1
  Electric Machine 1/2(EMPwrElec) -> [EMPwr1]
  Electric Machine 4/1(EMTrq) -> [EMTrq4]
  Electric Machine 3/1(EMTrq) -> [EMTrq3]
  Electric Machine 2/1(EMTrq) -> [EMTrq2]
  [EMTrq4] -> Vector Concatenate/4
  [EMTrq3] -> Vector Concatenate/3
  [EMTrq2] -> Vector Concatenate/2
  [EMTrq1] -> Vector Concatenate/1
  Electric Machine 1/1(EMTrq) -> [EMTrq1]
  Selector3/1 -> Electric Machine 4/1(EMTrqCmd)
  Selector1/1 -> Electric Machine 3/1(EMTrqCmd)
  Selector2/1 -> Electric Machine 2/1(EMTrqCmd)
  Vector Concatenate1/1 -> EMPwrElec/1  "EMPwrElec"
  Vector Concatenate/1 -> EMTrq/1  "EMTrq"
  Selector/1 -> Electric Machine 1/1(EMTrqCmd)
  EMTrqCmd/1 -> Selector/1, Selector3/1, Selector1/1, Selector2/1
  connections:
  Electric Machine 4/RConn1 -- Simscape Bus1/LConn4
  Electric Machine 3/RConn1 -- Simscape Bus1/LConn3
  EM/RConn1 -- Simscape Bus1/RConn1
  Electric Machine 2/RConn1 -- Simscape Bus1/LConn2
  Electric Machine 1/RConn1 -- Simscape Bus1/LConn1
  Electric Machine 3/LConn1 -- Electric Machine 1/LConn1 -- +/RConn1 -- Electric Machine 2/LConn1 -- Electric Machine 4/LConn1
  Electric Machine 3/LConn2 -- Electric Machine 1/LConn2 -- -/RConn1 -- Electric Machine 2/LConn2 -- Electric Machine 4/LConn2
  Connection Label1/LConn1 -- Simscape Bus/LConn1
  Connection Label3/LConn1 -- Simscape Bus/LConn2
  Simscape Bus/LConn3 -- Connection Label5/LConn1
  Connection Label/LConn1 -- Electric Machine 1/RConn2
  Connection Label2/LConn1 -- Electric Machine 2/RConn2
  ThrmEM/RConn1 -- Simscape Bus/RConn1
  Connection Label4/LConn1 -- Electric Machine 3/RConn2
  Simscape Bus/LConn4 -- Electric Machine 4/RConn2

== system SimscapePlantModels/Electrical System/Electrical System/Electric Machines/1EM/Electric Machine 1 ==
  EMTrqCmd : Inport
  Mapped EM : Subsystem  VariantControl=Mapped EM  ReferencedSubsystem=ElectricMachine1SSC
  + : PMIOPort  Side=Left
  - : PMIOPort  Port=2  Side=Left
  R : PMIOPort  Port=3  Side=Right
  H : PMIOPort  Port=4  Side=Right
  EMTrq : Outport  VectorParamsAs1DForOutWhenUnconnected=off
  EMPwrElec : Outport  Port=2  VectorParamsAs1DForOutWhenUnconnected=off

== system SimscapePlantModels/Electrical System/Electrical System/Electric Machines/2EM/Electric Machine 1 ==
  EMTrqCmd : Inport
  Mapped EM : Subsystem  VariantControl=Mapped EM  ReferencedSubsystem=ElectricMachine1SSC
  + : PMIOPort  Side=Left
  - : PMIOPort  Port=2  Side=Left
  R : PMIOPort  Port=3  Side=Right
  H : PMIOPort  Port=4  Side=Right
  EMTrq : Outport  VectorParamsAs1DForOutWhenUnconnected=off
  EMPwrElec : Outport  Port=2  VectorParamsAs1DForOutWhenUnconnected=off

== system SimscapePlantModels/Electrical System/Electrical System/Electric Machines/2EM/Electric Machine 2 ==
  EMTrqCmd : Inport
  Mapped EM : Subsystem  VariantControl=Mapped EM  ReferencedSubsystem=ElectricMachine2SSC
  + : PMIOPort  Side=Left
  - : PMIOPort  Port=2  Side=Left
  R : PMIOPort  Port=3  Side=Right
  H : PMIOPort  Port=4  Side=Right
  EMTrq : Outport  VectorParamsAs1DForOutWhenUnconnected=off
  EMPwrElec : Outport  Port=2  VectorParamsAs1DForOutWhenUnconnected=off

== system SimscapePlantModels/Electrical System/Electrical System/Electric Machines/3EM/Electric Machine 1 ==
  EMTrqCmd : Inport
  Mapped EM : Subsystem  VariantControl=Mapped EM  ReferencedSubsystem=ElectricMachine1SSC
  + : PMIOPort  Side=Left
  - : PMIOPort  Port=2  Side=Left
  R : PMIOPort  Port=3  Side=Right
  H : PMIOPort  Port=4  Side=Right
  EMTrq : Outport  VectorParamsAs1DForOutWhenUnconnected=off
  EMPwrElec : Outport  Port=2  VectorParamsAs1DForOutWhenUnconnected=off

== system SimscapePlantModels/Electrical System/Electrical System/Electric Machines/3EM/Electric Machine 2 ==
  EMTrqCmd : Inport
  Mapped EM : Subsystem  VariantControl=Mapped EM  ReferencedSubsystem=ElectricMachine2SSC
  + : PMIOPort  Side=Left
  - : PMIOPort  Port=2  Side=Left
  R : PMIOPort  Port=3  Side=Right
  H : PMIOPort  Port=4  Side=Right
  EMTrq : Outport  VectorParamsAs1DForOutWhenUnconnected=off
  EMPwrElec : Outport  Port=2  VectorParamsAs1DForOutWhenUnconnected=off

== system SimscapePlantModels/Electrical System/Electrical System/Electric Machines/3EM/Electric Machine 3 ==
  EMTrqCmd : Inport
  Mapped EM : Subsystem  VariantControl=Mapped EM  ReferencedSubsystem=ElectricMachine3SSC
  + : PMIOPort  Side=Left
  - : PMIOPort  Port=2  Side=Left
  R : PMIOPort  Port=3  Side=Right
  H : PMIOPort  Port=4  Side=Right
  EMTrq : Outport  VectorParamsAs1DForOutWhenUnconnected=off
  EMPwrElec : Outport  Port=2  VectorParamsAs1DForOutWhenUnconnected=off

== system SimscapePlantModels/Electrical System/Electrical System/Electric Machines/4EM/Electric Machine 1 ==
  EMTrqCmd : Inport
  Mapped EM : Subsystem  VariantControl=Mapped EM  ReferencedSubsystem=ElectricMachine1SSC
  + : PMIOPort  Side=Left
  - : PMIOPort  Port=2  Side=Left
  R : PMIOPort  Port=3  Side=Right
  H : PMIOPort  Port=4  Side=Right
  EMTrq : Outport  VectorParamsAs1DForOutWhenUnconnected=off
  EMPwrElec : Outport  Port=2  VectorParamsAs1DForOutWhenUnconnected=off

== system SimscapePlantModels/Electrical System/Electrical System/Electric Machines/4EM/Electric Machine 2 ==
  EMTrqCmd : Inport
  Mapped EM : Subsystem  VariantControl=Mapped EM  ReferencedSubsystem=ElectricMachine2SSC
  + : PMIOPort  Side=Left
  - : PMIOPort  Port=2  Side=Left
  R : PMIOPort  Port=3  Side=Right
  H : PMIOPort  Port=4  Side=Right
  EMTrq : Outport  VectorParamsAs1DForOutWhenUnconnected=off
  EMPwrElec : Outport  Port=2  VectorParamsAs1DForOutWhenUnconnected=off

== system SimscapePlantModels/Electrical System/Electrical System/Electric Machines/4EM/Electric Machine 3 ==
  EMTrqCmd : Inport
  Mapped EM : Subsystem  VariantControl=Mapped EM  ReferencedSubsystem=ElectricMachine3SSC
  + : PMIOPort  Side=Left
  - : PMIOPort  Port=2  Side=Left
  R : PMIOPort  Port=3  Side=Right
  H : PMIOPort  Port=4  Side=Right
  EMTrq : Outport  VectorParamsAs1DForOutWhenUnconnected=off
  EMPwrElec : Outport  Port=2  VectorParamsAs1DForOutWhenUnconnected=off

== system SimscapePlantModels/Electrical System/Electrical System/Electric Machines/4EM/Electric Machine 4 ==
  EMTrqCmd : Inport
  Mapped EM : Subsystem  VariantControl=Mapped EM  ReferencedSubsystem=ElectricMachine4SSC
  + : PMIOPort  Side=Left
  - : PMIOPort  Port=2  Side=Left
  R : PMIOPort  Port=3  Side=Right
  H : PMIOPort  Port=4  Side=Right
  EMTrq : Outport  VectorParamsAs1DForOutWhenUnconnected=off
  EMPwrElec : Outport  Port=2  VectorParamsAs1DForOutWhenUnconnected=off
